simulink model "lqr_sym"  (R2023b)
settings: Solver=VariableStepAuto  StartTime=0.0  StopTime=200  RelTol=1e-3
values from neighbouring files (symbols this model uses):
  A = [-p1-x2_eq -x1_eq; 0 -p2]    [WP2.m]    (also in lqr.m)
  B = [0; p3]    [WP2.m]    (also in lqr.m)
  equilibrium = [x1_eq,x2_eq].'    [lqr.m]
  K = [double(sol.k1) double(sol.k2)]    [WP2.m]    (also in lqr.m = lqr(sys, Qx, Qu))
  u_eq = 1.003    [WP2.m]    (also in lqr.m)
settings Model: Creator=kiraa  LastModifiedBy=david

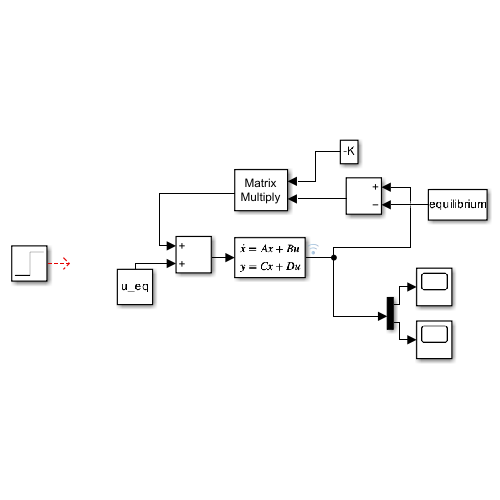
[thumbnail: Simulink's stored preview of the top-level diagram]
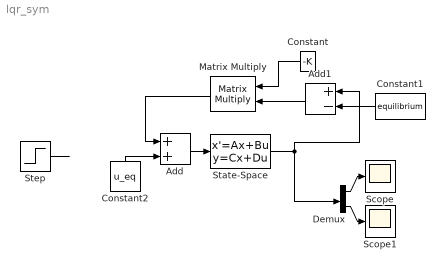
== system lqr_sym ==
  Add : Sum
  Add1 : Sum  Inputs=+-  InputSameDT=on  LockScale=on
  Constant : Constant  Value=-K  VectorParams1D=off
  Constant1 : Constant  Value=equilibrium  VectorParams1D=off
  Constant2 : Constant  Value=u_eq
  Demux : Demux  Outputs=2
  Matrix Multiply : Product  Multiplication=Matrix(*)
  Scope : Scope
  Scope1 : Scope
  State-Space : StateSpace  A=A  B=B  C=eye(2)  D=[0;0]  InitialCondition=[0,0]
  Step : Step  Before=u_eq  After=u_eq  SampleTime=0
  wires:
  Matrix Multiply/1 -> Add/1
  Constant/1 -> Matrix Multiply/1
  Demux/1 -> Scope/1
  Demux/2 -> Scope1/1
  Step/1 -> ?
  Constant1/1 -> Add1/2
  Add/1 -> State-Space/1
  State-Space/1 -> Add1/1, Demux/1
  Add1/1 -> Matrix Multiply/2
  Constant2/1 -> Add/2
